simulink model "Temp_Control_System_R2020a"  (R2023a)
settings: Solver=FixedStepAuto  StartTime=0.0  StopTime=10.0  MaxStep=1e-3  RelTol=1e-3
settings Model: Creator=hp  LastModifiedBy=hp
settings OptimizationCC: DefaultParameterBehavior=Inlined  UseDivisionForNetSlopeComputation=on  GainParamInheritBuiltInType=on  UseFloatMulNetSlope=on  InlineInvariantSignals=on  PassReuseOutputArgsAs=Individual arguments  ZeroExternalMemoryAtStartup=off  ZeroInternalMemoryAtStartup=off  NoFixptDivByZeroProtection=on  EfficientFloat2IntCast=on  LifeSpan=1  OptimizeBlockOrder=speed  DifferentSizesBufferReuse=on  EfficientTunableParamExpr=on
settings DebuggingCC: ParameterTunabilityLossMsg=error
settings HardwareCC: ProdLongLongMode=on
settings SFSimCC: MATLABDynamicMemAlloc=off
settings RTWCC: Description=Embedded Coder  SystemTargetFile=ert.tlc  TemplateMakefile=ert_default_tmf
settings CodeAppCC: ForceParamTrailComments=on  IgnoreCustomStorageClasses=off  OperatorAnnotations=on  SimulinkDataObjDesc=on  SFDataObjDesc=on  CustomSymbolStrGlobalVar=rt$N$M  CustomSymbolStrType=$N$M  CustomSymbolStrFcn=$N$M$F  CustomSymbolStrMacro=$N$M  InsertBlockDesc=on
settings ERTTargetCC: TargetLangStandard=C99 (ISO)  GenerateSampleERTMain=on  IncludeMdlTerminateFcn=off  CombineSignalStateStructs=on  SupportComplex=off  SupportContinuousTime=on  InlinedParameterPlacement=NonHierarchical  ERTCustomFileTemplate=example_file_process.tlc  ERTFilePackagingFormat=CompactWithDataFile

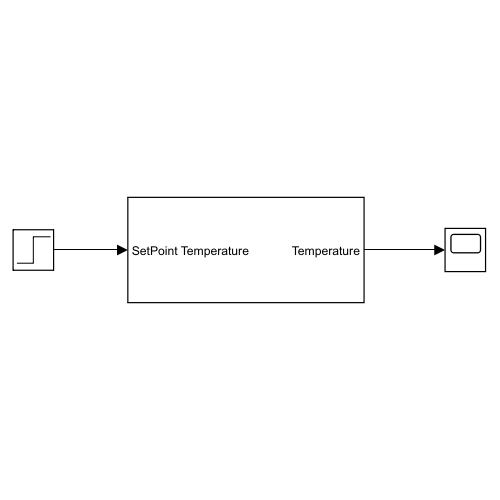
[thumbnail: Simulink's stored preview of the top-level diagram]
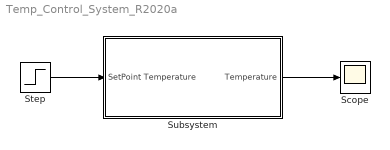
== system Temp_Control_System_R2020a ==
  Scope : Scope
  Step : Step  Time=2  Before=10  After=20  SampleTime=0
  Subsystem : Subsystem
  wires:
  Subsystem/1(Temperature) -> Scope/1
  Step/1 -> Subsystem/1(SetPoint Temperature)

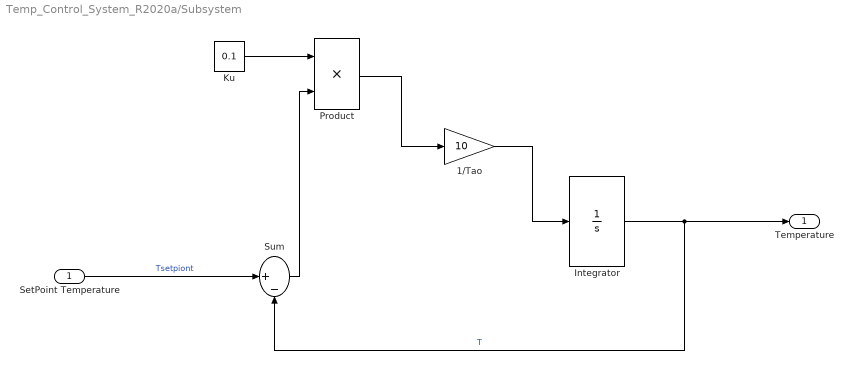
== system Temp_Control_System_R2020a/Subsystem ==
  SetPoint Temperature : Inport
  1/Tao : Gain  Gain=10
  Integrator : Integrator  InitialCondition=10
  Ku : Constant  Value=0.1
  Product : Product
  Sum : Sum  Inputs=|+-
  Temperature : Outport
  wires:
  Ku/1 -> Product/1
  SetPoint Temperature/1 -> Sum/1  "Tsetpiont"
  Integrator/1 -> Sum/2, Temperature/1  "T"
  Sum/1 -> Product/2
  Product/1 -> 1/Tao/1
  1/Tao/1 -> Integrator/1
